simulink model "PenduloRotativoSim"  (R2025a)
settings: Solver=VariableStepAuto  StartTime=0.0  StopTime=20  FixedStep=1e-4  RelTol=1e-3  EnableMultiTasking=on
StopFcn:
  | send_to_visualizer(out.theta1_out, out.theta2_out)
values from neighbouring files (symbols this model uses):
  d = sig.signals.values(:)    [send_to_visualizer.m]
  esc_amp = 0.05    [preparaSimulacao.m]
  esc_gain = 500    [preparaSimulacao.m]
  k_init = 0.3    [preparaSimulacao.m]
  mod_freq = 2*pi*15    (= 94.2477796077)    [preparaSimulacao.m]
  w_hf = mod_freq/5    (= 18.8495559215)    [preparaSimulacao.m]
  x_ic = [deg2rad(170); 0;]    [preparaSimulacao.m]
  xp_ic = [0;0]    [preparaSimulacao.m]
undefined symbols (not defined in the file or in its folder): den, DiscIntNeverNeededParam, Jh, Jr, K, L, Mh, Mr, num, Ts
settings Model: SimulationMode=external  ExtModeTrigDuration=10000  Creator=aluno.engenharia  LastModifiedBy=gabri
settings SolverCC: AlgebraicLoopSolver=TrustRegion  PositivePriorityOrder=on
settings DebuggingCC: UnconnectedInputMsg=warning  UnconnectedOutputMsg=warning  UnconnectedLineMsg=warning
settings ModelReferenceCC: EnableRefExpFcnMdlSchedulingChecks=on
settings SFSimCC: CustomCodeUndefinedFunction=UseInterfaceOnly
settings RTWCC: SystemTargetFile=quarc_win64.tlc  TemplateMakefile=quarc_default_tmf  GPUComputeCapability=3.5  Description=QUARC Win64 Target
settings STFCustomTargetCC: SystemTargetFile=quarc_win64.tlc  TargetPreCompLibLocation=C:\PROGRA~3\QUARC\lib\2019a\win64\release  TargetLangStandard=C99 (ISO)  MultiwordLength=2048.0  DynamicStringBufferSize=256.0  ConcurrentExecutionCompliant=on  DownloadToTarget=on  StopOnOverrun=off  Debug=off
settings GRTTargetCC: ExtMode=on  ExtModeMexFile=quarc_comm  TargetPreCompLibLocation=C:\PROGRA~3\QUARC\lib\2019a\win64\release  ParMdlRefBuildCompliant=off  CompOptLevelCompliant=off  CombineOutputUpdateFcns=off  MatFileLogging=off  CPPClassGenCompliant=off  GRTInterface=on  UseToolchainInfoCompliant=off

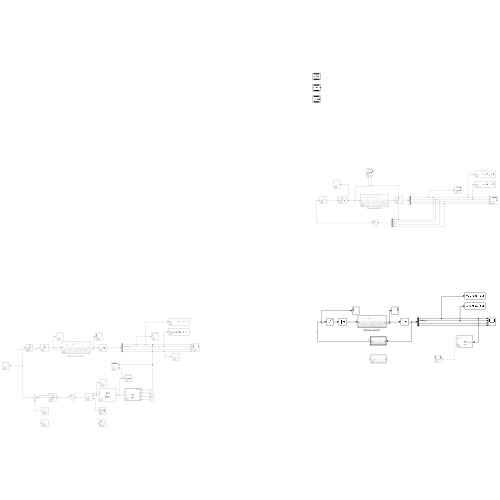
[thumbnail: Simulink's stored preview of the top-level diagram]
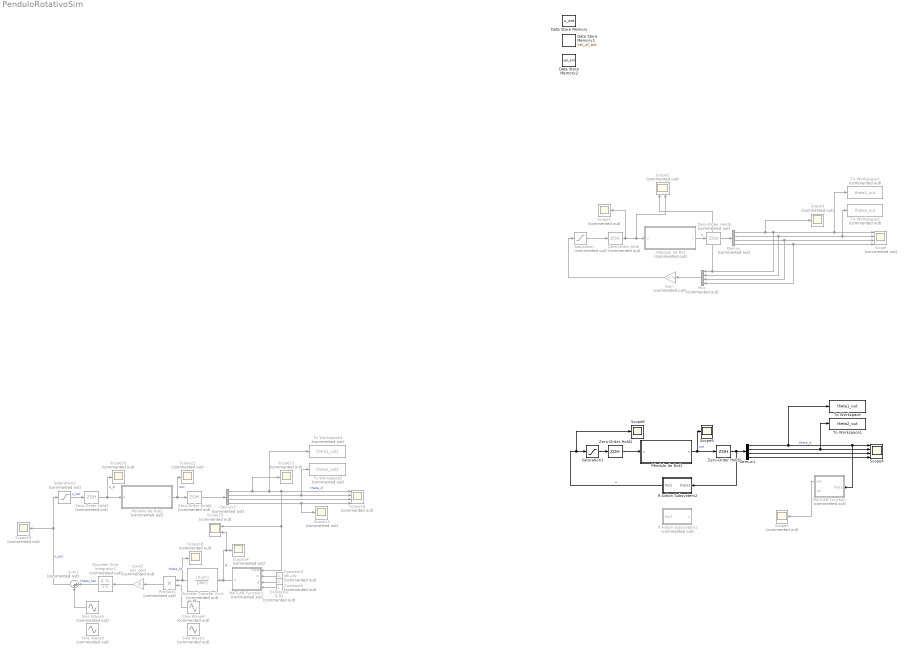
== system PenduloRotativoSim ==
  note: w_hf
  Constant3 : Constant  Commented=on  Value=Mh+Mr
  Constant4 : Constant  Commented=on  Value=9.81
  Constant5 : Constant  Commented=on  Value=L
  Data Store Memory : DataStoreMemory  DataStoreName=u_ant  ShowAdditionalParam=off  OutDataTypeStr=double
  Data Store Memory1 : DataStoreMemory  DataStoreName=vel_uf_ant  ReadBeforeWriteMsg=warning  WriteAfterWriteMsg=warning  WriteAfterReadMsg=warning  ShowAdditionalParam=off  OutDataTypeStr=double
  Data Store Memory2 : DataStoreMemory  DataStoreName=vel_ant  ReadBeforeWriteMsg=warning  WriteAfterWriteMsg=warning  WriteAfterReadMsg=warning  ShowAdditionalParam=off  OutDataTypeStr=double
  Demux : Demux  Commented=on
  Demux1 : Demux
  Demux2 : Demux  Commented=on
  Discrete Transfer Fcn1 : DiscreteTransferFcn  Commented=on  Numerator=[num]  Denominator=[den]
  Discrete-Time Integrator1 : DiscreteIntegrator  Commented=on  SampleTime=-1  ICPrevOutput=DiscIntNeverNeededParam  ICPrevScaledInput=DiscIntNeverNeededParam
  Gain : Gain  Commented=on  Gain=-K  Multiplication=Matrix(K*u)
  Gain2 : Gain  Commented=on  Gain=esc_gain
  If Action Subsystem1 : Subsystem  Commented=on  TreatAsAtomicUnit=on
  If Action Subsystem2 : Subsystem  TreatAsAtomicUnit=on
  MATLAB Function : MATLAB Function  Commented=on  TreatAsAtomicUnit=on
  MATLAB Function1 : MATLAB Function  Commented=on  TreatAsAtomicUnit=on
  Mux : Mux  Commented=on
  Product1 : Product  Commented=on
  Pêndulo de Rot : Subsystem  Commented=on
  Pêndulo de Rot1 : Subsystem
  Pêndulo de Rot2 : Subsystem  Commented=on
  Saturation : Saturate  Commented=on  UpperLimit=1  LowerLimit=-1
  Saturation1 : Saturate  UpperLimit=1  LowerLimit=-1
  Saturation2 : Saturate  Commented=on  UpperLimit=12  LowerLimit=-12
  Scope : Scope  Commented=on  NumInputPorts=4
      settings: ActiveDisplayYMinimum=-0.098888624772432612  ActiveDisplayYMaximum=0.3018758336404363
  Scope{1,3,5,13..14,17..21} (10 alike) : Scope  Commented=on
      Scope1 settings: ActiveDisplayYMinimum=0.9  ActiveDisplayYMaximum=1.1  DataLoggingVariableName=ScopeData3
      Scope13 settings: ActiveDisplayYMinimum=-16.31486477328804  ActiveDisplayYMaximum=9.08544811182352  DataLoggingVariableName=ScopeData15
      Scope14 settings: ActiveDisplayYMinimum=-0.9244908487241017  ActiveDisplayYMaximum=0.10098357051691505  DataLoggingVariableName=ScopeData16
      Scope17 settings: ActiveDisplayYMinimum=2.9767729826768266  ActiveDisplayYMaximum=4.1753725629581435  DataLoggingVariableName=ScopeData19
      Scope18 settings: ActiveDisplayYMinimum=-1  ActiveDisplayYMaximum=1  DataLoggingVariableName=ScopeData20
      Scope19 settings: ActiveDisplayYMinimum=-0.14582093757057762  ActiveDisplayYMaximum=0.18698042473953164  DataLoggingVariableName=ScopeData21
      Scope20 settings: ActiveDisplayYMinimum=-1  ActiveDisplayYMaximum=1  DataLoggingVariableName=ScopeData22
      Scope21 settings: ActiveDisplayYMinimum=0.36169099404350114  ActiveDisplayYMaximum=3.9175028405366232  DataLoggingVariableName=ScopeData23
      Scope3 settings: ActiveDisplayYMinimum=-0.29202531249135588  ActiveDisplayYMaximum=6.0864290081646626  DataLoggingVariableName=ScopeData5
      Scope5 settings: ActiveDisplayYMinimum=-0.12499999999999997  ActiveDisplayYMaximum=1.125  DataLoggingVariableName=ScopeData9
  Scope15 : Scope  Commented=on  NumInputPorts=2
      settings: ActiveDisplayYMinimum=4.2300428343533376  ActiveDisplayYMaximum=5.2203237501157735  DataLoggingVariableName=ScopeData17
  Scope16 : Scope  Commented=on  NumInputPorts=4
      settings: ActiveDisplayYMinimum=-0.537870966208293  ActiveDisplayYMaximum=5.7135033218718032  DataLoggingVariableName=ScopeData18
  Scope2 : Scope  Commented=on  NumInputPorts=2
      settings: ActiveDisplayYMinimum=-13.721058256878093  ActiveDisplayYMaximum=11.6029022738507  DataLoggingVariableName=ScopeData4
  Scope4 : Scope  NumInputPorts=4
      settings: ActiveDisplayYMinimum=-99.926748678400074  ActiveDisplayYMaximum=18.030278546190754  DataLoggingVariableName=ScopeData6
  Scope8 : Scope
      settings: ActiveDisplayYMinimum=-2460.238292726006  ActiveDisplayYMaximum=1645.9640823338532  DataLoggingVariableName=ScopeData10
  Scope9 : Scope
      settings: ActiveDisplayYMinimum=0.36169099404350114  ActiveDisplayYMaximum=3.9175028405366232  DataLoggingVariableName=ScopeData11
  Sine Wave1 : Sin  Commented=on  SineType=Sample based  Frequency=mod_freq  Samples=round(2*pi/(mod_freq*2e-4))  SampleTime=0.0002
  Sine Wave3 : Sin  Commented=on  SineType=Sample based  Amplitude=esc_amp  Frequency=mod_freq  Samples=round(2*pi/(mod_freq*2e-4))  SampleTime=0.0002
  Sine Wave4 : Sin  Commented=on  Frequency=mod_freq  Samples=round(2*pi/(mod_freq*2e-4))  SampleTime=0
  Sine Wave5 : Sin  Commented=on  Amplitude=esc_amp  Frequency=mod_freq  Samples=round(2*pi/(mod_freq*2e-4))  SampleTime=0
  Sum1 : Sum  Commented=on  Inputs=|++
  To Workspace : ToWorkspace  VariableName=theta1_out  SaveFormat=Timeseries  SampleTime=-1
  To Workspace1 : ToWorkspace  VariableName=theta2_out  SaveFormat=Timeseries  SampleTime=-1
  To Workspace2 : ToWorkspace  Commented=on  VariableName=theta1_out  SaveFormat=Timeseries  SampleTime=-1
  To Workspace3 : ToWorkspace  Commented=on  VariableName=theta2_out  SaveFormat=Timeseries  SampleTime=-1
  To Workspace4 : ToWorkspace  Commented=on  VariableName=theta1_out1  SaveFormat=Timeseries  SampleTime=-1
  To Workspace5 : ToWorkspace  Commented=on  VariableName=theta2_out1  SaveFormat=Timeseries  SampleTime=-1
  Zero-Order Hold{,3..5} (4 alike) : ZeroOrderHold  Commented=on  SampleTime=Ts
  Zero-Order Hold1 : ZeroOrderHold  SampleTime=Ts
  Zero-Order Hold2 : ZeroOrderHold  SampleTime=Ts
  wires:
  Gain/1 -> Saturation/1
  Demux/2 -> Mux/2, To Workspace3/1, Scope/2
  Demux/3 -> Scope/3, Mux/3
  Demux/4 -> Scope/4, Mux/4
  Saturation/1 -> Zero-Order Hold/1
  Pêndulo de Rot/1(x) -> Zero-Order Hold5/1  "x"
  Demux/1 -> Scope3/1, Scope2/1, Mux/1, To Workspace2/1, Scope/1
  Mux/1 -> Gain/1
  Zero-Order Hold/1 -> Scope2/2, Pêndulo de Rot/1(u), Scope1/1
  Demux1/3 -> Scope4/3
  Demux1/4 -> Scope4/4
  Demux1/1 -> To Workspace/1, MATLAB Function/1(theta), Scope4/1  "theta_d"
  Demux1/2 -> To Workspace1/1, Scope4/2
  Pêndulo de Rot1/1(x) -> Scope9/1, Zero-Order Hold2/1  "out"
  Demux2/2 -> To Workspace5/1, Scope16/2
  Demux2/3 -> Scope16/3
  MATLAB Function1/1(U) -> Scope15/2, Scope14/1, Discrete Transfer Fcn1/1  "U"
  Constant4/1 -> MATLAB Function1/3(g)
  Product1/1 -> Gain2/1
  Constant3/1 -> MATLAB Function1/2(m)
  Pêndulo de Rot2/1(x) -> Scope21/1, Zero-Order Hold4/1  "out"
  Constant5/1 -> MATLAB Function1/4(l)
  Sine Wave4/1 -> Product1/2
  Demux2/1 -> Scope17/1, To Workspace4/1, MATLAB Function1/1(theta), Scope15/1, Scope16/1  "theta_d"
  Sum1/1 -> Saturation2/1, Scope19/1  "u_esc"
  Demux2/4 -> Scope13/1, Scope16/4
  Zero-Order Hold4/1 -> Demux2/1
  Sine Wave5/1 -> Sum1/2
  Discrete-Time Integrator1/1 -> Sum1/1  "theta_hat"
  Discrete Transfer Fcn1/1 -> Scope18/1, Product1/1  "theta_hf"
  Saturation2/1 -> Zero-Order Hold3/1  "u_sat"
  Zero-Order Hold3/1 -> Scope20/1, Pêndulo de Rot2/1(u)  "u_d"
  Gain2/1 -> Discrete-Time Integrator1/1
  MATLAB Function/1(esc) -> Scope5/1
  Zero-Order Hold1/1 -> Pêndulo de Rot1/1(u)
  Zero-Order Hold2/1 -> If Action Subsystem2/1(theta1), Demux1/1
  Zero-Order Hold5/1 -> Demux/1
  If Action Subsystem2/1(Out1) -> Saturation1/1, Scope8/1  "u"
  Saturation1/1 -> Zero-Order Hold1/1

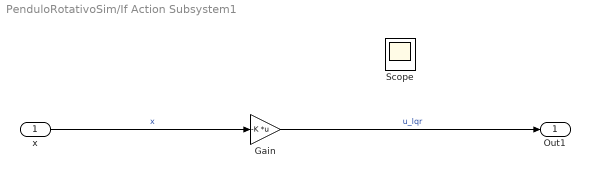
== system PenduloRotativoSim/If Action Subsystem1 ==
  x : Inport
  Gain : Gain  Gain=-K  Multiplication=Matrix(K*u)
  Scope : Scope
      settings: ActiveDisplayYMinimum=-4.4404726516390376  ActiveDisplayYMaximum=69.774089352779029  DataLoggingVariableName=ScopeData12
  Out1 : Outport
  wires:
  x/1 -> Gain/1  "x"
  Gain/1 -> Out1/1  "u_lqr"

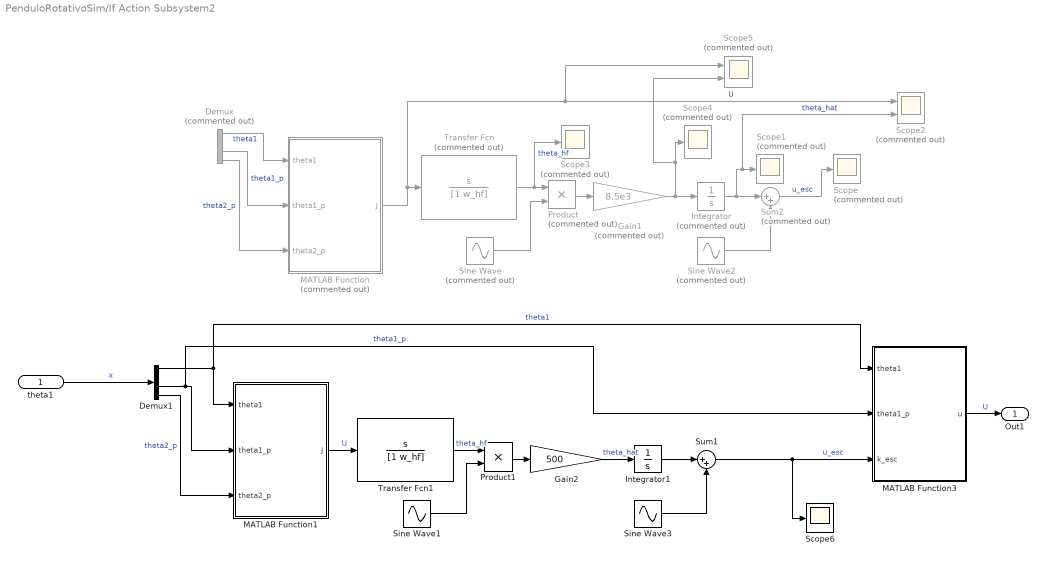
== system PenduloRotativoSim/If Action Subsystem2 ==
  theta1 : Inport
  Demux : Demux  Commented=on
  Demux1 : Demux
  Gain1 : Gain  Commented=on  Gain=8.5e3
  Gain2 : Gain  Gain=500
  Integrator : Integrator  Commented=on
  Integrator1 : Integrator  InitialCondition=k_init
  MATLAB Function : MATLAB Function  Commented=on  TreatAsAtomicUnit=on
  MATLAB Function1 : MATLAB Function  TreatAsAtomicUnit=on
  MATLAB Function3 : MATLAB Function  TreatAsAtomicUnit=on
  Product : Product  Commented=on
  Product1 : Product
  Scope{,1,3..4} (4 alike) : Scope  Commented=on
      Scope settings: ActiveDisplayYMinimum=-1  ActiveDisplayYMaximum=1  DataLoggingVariableName=ScopeData13
      Scope1 settings: ActiveDisplayYMinimum=-3.2058024078374254  ActiveDisplayYMaximum=-0.96848992459031114  DataLoggingVariableName=ScopeData14
      Scope3 settings: ActiveDisplayYMinimum=-0.021431987322528941  ActiveDisplayYMaximum=0.013260172312204901  DataLoggingVariableName=ScopeData8
      Scope4 settings: ActiveDisplayYMinimum=-4.2044520300748793  ActiveDisplayYMaximum=8.6338341823384948  DataLoggingVariableName=ScopeData24
  Scope2 : Scope  Commented=on  NumInputPorts=2
      settings: ActiveDisplayYMinimum=-3.3789414590063629  ActiveDisplayYMaximum=0.054695354489563641  DataLoggingVariableName=ScopeData7
  Scope5 : Scope  Commented=on  NumInputPorts=2
      settings: ActiveDisplayYMinimum=-0.24757580720707464  ActiveDisplayYMaximum=0.58612214942196117  DataLoggingVariableName=ScopeData25
  Scope6 : Scope
      settings: ActiveDisplayYMinimum=-1  ActiveDisplayYMaximum=1  DataLoggingVariableName=ScopeData26
  Sine Wave : Sin  Commented=on  Frequency=mod_freq  Samples=round(2*pi/(mod_freq*2e-4))  SampleTime=0
  Sine Wave1 : Sin  Frequency=mod_freq  Samples=round(2*pi/(mod_freq*2e-4))  SampleTime=0
  Sine Wave2 : Sin  Commented=on  Amplitude=0.05  Frequency=mod_freq  Samples=round(2*pi/(mod_freq*2e-4))  SampleTime=0
  Sine Wave3 : Sin  Amplitude=esc_amp  Frequency=mod_freq  Samples=round(2*pi/(mod_freq*2e-4))  SampleTime=0
  Sum1 : Sum  Inputs=|++
  Sum2 : Sum  Commented=on  Inputs=|++
  Transfer Fcn : TransferFcn  Commented=on  Numerator=[1 0]  Denominator=[1 w_hf]
  Transfer Fcn1 : TransferFcn  Numerator=[1 0]  Denominator=[1 w_hf]
  Out1 : Outport
  wires:
  Demux/1 -> MATLAB Function/1(theta1)  "theta1"
  Demux/3 -> MATLAB Function/2(theta1_p)  "theta1_p"
  Gain1/1 -> Scope4/1, Scope5/2, Integrator/1
  Demux/4 -> MATLAB Function/3(theta2_p)  "theta2_p"
  Product/1 -> Gain1/1
  MATLAB Function/1(J) -> Scope5/1, Scope2/1, Transfer Fcn/1  "U"
  Integrator/1 -> Scope2/2, Scope1/1, Sum2/1  "theta_hat"
  Transfer Fcn/1 -> Scope3/1, Product/1  "theta_hf"
  Sum2/1 -> Scope/1  "u_esc"
  Sine Wave/1 -> Product/2
  Sine Wave2/1 -> Sum2/2
  Product1/1 -> Gain2/1
  Demux1/4 -> MATLAB Function1/3(theta2_p)  "theta2_p"
  Demux1/3 -> MATLAB Function3/2(theta1_p), MATLAB Function1/2(theta1_p)  "theta1_p"
  Sine Wave1/1 -> Product1/2
  Sum1/1 -> Scope6/1, MATLAB Function3/3(k_esc)  "u_esc"
  Gain2/1 -> Integrator1/1  "theta_hat"
  Transfer Fcn1/1 -> Product1/1  "theta_hf"
  theta1/1 -> Demux1/1  "x"
  Demux1/1 -> MATLAB Function3/1(theta1), MATLAB Function1/1(theta1)  "theta1"
  Sine Wave3/1 -> Sum1/2
  MATLAB Function1/1(J) -> Transfer Fcn1/1  "U"
  Integrator1/1 -> Sum1/1
  MATLAB Function3/1(u) -> Out1/1  "U"

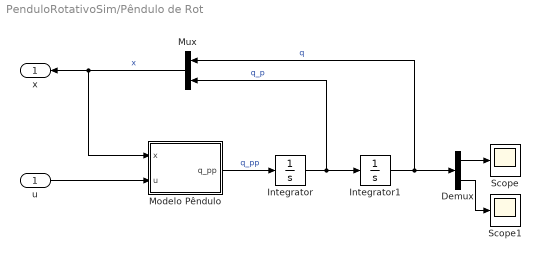
== system PenduloRotativoSim/Pêndulo de Rot ==
  u : Inport
  Demux : Demux  Outputs=2
  Integrator : Integrator  InitialCondition=xp_ic
  Integrator1 : Integrator  InitialCondition=x_ic
  Modelo Pêndulo : MATLAB Function  TreatAsAtomicUnit=on
  Mux : Mux  Inputs=2
  Scope : Scope
      settings: ActiveDisplayYMinimum=-4.469489019623639  ActiveDisplayYMaximum=6.9006379196709613
  Scope1 : Scope
      settings: ActiveDisplayYMinimum=-4.469489019623639  ActiveDisplayYMaximum=6.9006379196709613  DataLoggingVariableName=ScopeData2
  x : Outport
  wires:
  Mux/1 -> x/1, Modelo Pêndulo/1(x)  "x"
  Modelo Pêndulo/1(q_pp) -> Integrator/1  "q_pp"
  u/1 -> Modelo Pêndulo/2(u)
  Integrator/1 -> Mux/2, Integrator1/1  "q_p"
  Integrator1/1 -> Mux/1, Demux/1  "q"
  Demux/1 -> Scope/1
  Demux/2 -> Scope1/1

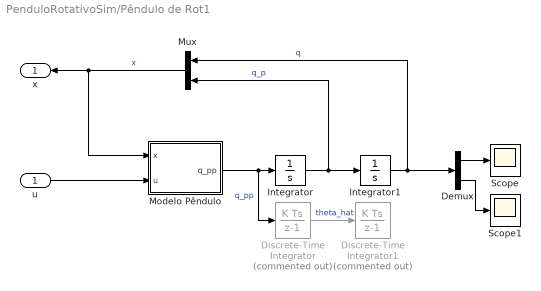
== system PenduloRotativoSim/Pêndulo de Rot1 ==
  u : Inport
  Demux : Demux  Outputs=2
  Discrete-Time Integrator : DiscreteIntegrator  Commented=on  InitialCondition=xp_ic  SampleTime=-1  ICPrevOutput=DiscIntNeverNeededParam  ICPrevScaledInput=DiscIntNeverNeededParam
  Discrete-Time Integrator1 : DiscreteIntegrator  Commented=on  InitialCondition=x_ic  SampleTime=-1  ICPrevOutput=DiscIntNeverNeededParam  ICPrevScaledInput=DiscIntNeverNeededParam
  Integrator : Integrator  InitialCondition=xp_ic
  Integrator1 : Integrator  InitialCondition=x_ic
  Modelo Pêndulo : MATLAB Function  TreatAsAtomicUnit=on
  Mux : Mux  Inputs=2
  Scope : Scope
      settings: ActiveDisplayYMinimum=-4.469489019623639  ActiveDisplayYMaximum=6.9006379196709613
  Scope1 : Scope
      settings: ActiveDisplayYMinimum=-4.469489019623639  ActiveDisplayYMaximum=6.9006379196709613  DataLoggingVariableName=ScopeData2
  x : Outport
  wires:
  Mux/1 -> x/1, Modelo Pêndulo/1(x)  "x"
  Modelo Pêndulo/1(q_pp) -> Integrator/1, Discrete-Time Integrator/1  "q_pp"
  u/1 -> Modelo Pêndulo/2(u)
  Demux/1 -> Scope/1
  Demux/2 -> Scope1/1
  Discrete-Time Integrator/1 -> Discrete-Time Integrator1/1  "theta_hat"
  Integrator/1 -> Mux/2, Integrator1/1  "q_p"
  Integrator1/1 -> Demux/1, Mux/1  "q"

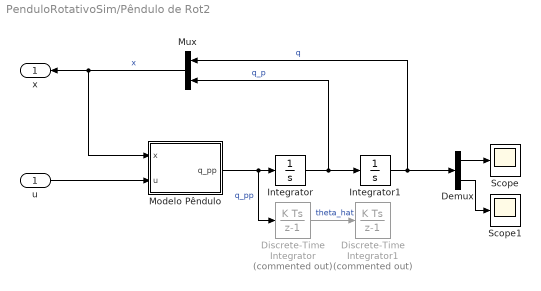
== system PenduloRotativoSim/Pêndulo de Rot2 ==
  u : Inport
  Demux : Demux  Outputs=2
  Discrete-Time Integrator : DiscreteIntegrator  Commented=on  InitialCondition=xp_ic  SampleTime=-1  ICPrevOutput=DiscIntNeverNeededParam  ICPrevScaledInput=DiscIntNeverNeededParam
  Discrete-Time Integrator1 : DiscreteIntegrator  Commented=on  InitialCondition=x_ic  SampleTime=-1  ICPrevOutput=DiscIntNeverNeededParam  ICPrevScaledInput=DiscIntNeverNeededParam
  Integrator : Integrator  InitialCondition=xp_ic
  Integrator1 : Integrator  InitialCondition=x_ic
  Modelo Pêndulo : MATLAB Function  TreatAsAtomicUnit=on
  Mux : Mux  Inputs=2
  Scope : Scope
      settings: ActiveDisplayYMinimum=-4.469489019623639  ActiveDisplayYMaximum=6.9006379196709613
  Scope1 : Scope
      settings: ActiveDisplayYMinimum=-4.469489019623639  ActiveDisplayYMaximum=6.9006379196709613  DataLoggingVariableName=ScopeData2
  x : Outport
  wires:
  Mux/1 -> x/1, Modelo Pêndulo/1(x)  "x"
  Modelo Pêndulo/1(q_pp) -> Integrator/1, Discrete-Time Integrator/1  "q_pp"
  u/1 -> Modelo Pêndulo/2(u)
  Demux/1 -> Scope/1
  Demux/2 -> Scope1/1
  Discrete-Time Integrator/1 -> Discrete-Time Integrator1/1  "theta_hat"
  Integrator/1 -> Mux/2, Integrator1/1  "q_p"
  Integrator1/1 -> Demux/1, Mux/1  "q"

== matlab function PenduloRotativoSim/Pêndulo de Rot/Modelo Pêndulo ==
  data: x input; q_pp output; u input
function q_pp = fcn(x,u)

th0_  = x(1);
th1_ = x(2);
th0_p  = x(3);
th1_p = x(4);


% Matrizes modelo forma geral (reduziada)
M = function_M_Rot();
V = function_V_Rot(th0_p, th1_p);
G = function_G_Rot(th0_);
P = function_P_Rot();

q_pp = M^-1*(P*u-V-G);

== matlab function PenduloRotativoSim/Pêndulo de Rot1/Modelo Pêndulo ==
  data: x input; q_pp output; u input
function q_pp = fcn(x,u)

th0_  = x(1);
th1_ = x(2);
th0_p  = x(3);
th1_p = x(4);


% Matrizes modelo forma geral (reduzida)
M = function_M_Rot();
V = function_V_Rot(th0_p, th1_p);
G = function_G_Rot(th0_);
P = function_P_Rot();

q_pp = M^-1*(P*u-V-G);

== matlab function PenduloRotativoSim/MATLAB Function ==
  data: theta input; esc output; lqr output
function [esc,lqr]= fcn(theta)
    % Wrap to [-pi, pi] — always gives shortest angle to upright (0)
    theta = atan2(sin(theta), cos(theta));
    esc = abs(theta) < deg2rad(20);
    lqr = not(esc);
end

== matlab function PenduloRotativoSim/MATLAB Function1 ==
  data: theta input; U output; m input; g input; l input
function U = fcn(theta, m, g, l)


U = m*g*l*(cos(theta) - 1);

== matlab function PenduloRotativoSim/Pêndulo de Rot2/Modelo Pêndulo ==
  data: x input; q_pp output; u input
function q_pp = fcn(x,u)

th0_  = x(1);
th1_ = x(2);
th0_p  = x(3);
th1_p = x(4);


% Matrizes modelo forma geral (reduzida)
M = function_M_Rot();
V = function_V_Rot(th0_p, th1_p);
G = function_G_Rot(th0_);
P = function_P_Rot();

q_pp = M^-1*(P*u-V-G);

== matlab function PenduloRotativoSim/If Action Subsystem2/MATLAB Function1 ==
  data: theta1 input; theta1_p input; theta2_p input; J output; Mr parameter; Mh parameter; L parameter; d parameter; Jh parameter; Jr parameter
function J = cost_function(theta1, theta1_p, theta2_p, Mr, Mh, L, d, Jh, Jr)
    % Pendulum-only inertia (no wheel coupling terms)
    J_pend = Mr*L^2 + Jh;
    Vg = (Mh*L + Mr*d)*9.81;
    
    % Pendulum-only mechanical energy
    KE_pend = 0.5 * J_pend * theta1_p^2;
    PE = Vg * cos(theta1);
    E_pend = KE_pend + PE;
    
    % Target: pendulum energy at upright rest
    E_target = Vg;
    
    J = -(E_pend - E_target)^2;
end

== matlab function PenduloRotativoSim/If Action Subsystem2/MATLAB Function ==
  data: theta1 input; theta1_p input; theta2_p input; J output; Mr parameter; Mh parameter; L parameter; d parameter; Jh parameter; Jr parameter
function J = cost_function(theta1, theta1_p, theta2_p, Mr, Mh, L, d, Jh, Jr)
    % Pendulum-only inertia (no wheel coupling terms)
    J_pend = Mr*L^2 + Jh;
    Vg = (Mh*L + Mr*d)*9.81;
    
    % Pendulum-only mechanical energy
    KE_pend = 0.5 * J_pend * theta1_p^2;
    PE = Vg * cos(theta1);
    E_pend = KE_pend + PE;
    
    % Target: pendulum energy at upright rest
    E_target = Vg;
    
    J = -(E_pend - E_target)^2;
end

== matlab function PenduloRotativoSim/If Action Subsystem2/MATLAB Function3 ==
  data: theta1 input; theta1_p input; Mr parameter; Mh parameter; L parameter; d parameter; Jh parameter; k_esc input; u output
function u = energy_pump(theta1, theta1_p, Mr, Mh, L, d, Jh, k_esc)
    % Parameters (set as block parameters from workspace)
    J_pend = Mr*L^2 + Jh;
    Vg = (Mh*L + Mr*d)*9.81;
    
    % Pendulum-only energy
    KE_pend = 0.5 * J_pend * theta1_p^2;
    PE = Vg * cos(theta1);
    E_pend = KE_pend + PE;
    
    E_target = Vg;
    
    % Energy pumping with ESC-tuned gain
    u = k_esc * sign(theta1_p) * sign(E_target - E_pend);
    
end
